simulink model "WF_onshore"  (R2024a)
settings: Solver=VariableStepAuto  StartTime=0  StopTime=0.9  RelTol=1e-3
values from neighbouring files (symbols this model uses):
  cvtr = initialize_NR_VSC_GF(cvtr)    [NR_steadystate_VSC_GF.m]    (also in WF_onshore_SSO_GFL.m = setfield(cvtr,'parameters', p_vary.name,p_vary.val(i)); WF_physical_param_offshore_supersynchronous.m = setfield(cvtr,'parameters', p_vary.name,p_vary.val(i)); WF_physical_param_onshore_SSO_020625.m = setfield(cvtr,'parameters', p_vary.name,p_vary.val(i)); impedance_WT_blackbox.m = base_values(cvtr))
  cvtr1 = cvtr_agg    [WF_physical_param_onshore_SSO_020625.m]
  enable_pll = 1    [impedance_WT_agg.m]    (also in initialize_WT_agg.m; initialize_WT_default_gfl.m; initialize_WT_default_offshore_super.m)
  f1 = 50    [WF_onshore_SSO_GFL.m]    (also in WF_physical_param_offshore_supersynchronous.m; WF_physical_param_onshore_SSO_020625.m; initialize_params_agg.m)
  i = 1    [WF_physical_param_offshore_supersynchronous.m]    (also in WF_physical_param_onshore_SSO_020625.m)
  L = inv(R)    [participation_factors_VSC_GF.m]
  l_OH = 0.2    [WF_onshore_SSO_GFL.m]    (also in WF_physical_param_offshore_supersynchronous.m = 0.1; WF_physical_param_onshore_SSO_020625.m = 0.1; initialize_params_agg.m = 0.1)
  l_tf_wf = tf_params(2,2)    [IM_WF_agg.m]    (also in WF_onshore_SSO_GFL.m = 0.05; WF_physical_param_offshore_supersynchronous.m = 0.05; WF_physical_param_onshore_SSO_020625.m = 0.05; initialize_params_agg.m = 0.05)
  l_tf_wt = tf_params(1,2)    [IM_WF_agg.m]    (also in WF_onshore_SSO_GFL.m = 0.0392; WF_physical_param_offshore_supersynchronous.m = 0.0392; WF_physical_param_onshore_SSO_020625.m = 0.0392; initialize_params_agg.m = 0.0392)
  Lg = p_vary(i)*((Z_b_G/(2*pi*f1)))    [WF_onshore_SSO_GFL.m]    (also in WF_physical_param_offshore_supersynchronous.m; WF_physical_param_onshore_SSO_020625.m; initialize_params_agg.m = 0.1*((Z_b_G/(2*pi*f1))))
  Lg1 = Lg    [WF_physical_param_offshore_supersynchronous.m]    (also in WF_physical_param_onshore_SSO_020625.m)
  Lg2 = Lg    [WF_physical_param_offshore_supersynchronous.m]    (also in WF_physical_param_onshore_SSO_020625.m)
  r_OH = 0.02    [WF_onshore_SSO_GFL.m]    (also in WF_physical_param_offshore_supersynchronous.m = 0.01; WF_physical_param_onshore_SSO_020625.m = 0.01; initialize_params_agg.m)
  r_tf_wf = tf_params(2,1)    [IM_WF_agg.m]    (also in WF_onshore_SSO_GFL.m = 0.005; WF_physical_param_offshore_supersynchronous.m = 0.005; WF_physical_param_onshore_SSO_020625.m = 0.005; initialize_params_agg.m = 0.005)
  r_tf_wt = tf_params(1,1)    [IM_WF_agg.m]    (also in WF_onshore_SSO_GFL.m = 0.0056; WF_physical_param_offshore_supersynchronous.m = 0.0056; WF_physical_param_onshore_SSO_020625.m = 0.0056; initialize_params_agg.m = 0.0056)
  Rg = rg*Z_b_G    [WF_onshore_SSO_GFL.m]    (also in WF_physical_param_offshore_supersynchronous.m; WF_physical_param_onshore_SSO_020625.m; initialize_params_agg.m = 0.01*Z_b_G)
  Sb_WF = (3*1)*5e6    (= 15000000)    [WF_onshore_SSO_GFL.m]    (also in WF_physical_param_offshore_supersynchronous.m; WF_physical_param_onshore_SSO_020625.m; impedance_WT_blackbox.m = n_t*Sb_WT; initialize_params_agg.m = 1000000000)
  Sb_WT = 5e6    (= 5000000)    [IM_WF.m]    (also in WF_onshore_SSO_GFL.m; WF_physical_param_offshore_supersynchronous.m; WF_physical_param_onshore_SSO_020625.m; initialize_params_agg.m)
  selector_current_reference = 3    [impedance_WT_agg.m]    (also in initialize_WT_agg.m; initialize_WT_default_gfl.m; initialize_WT_default_offshore_super.m)
  selector_omega_reference = 1    [impedance_WT_agg.m]    (also in initialize_WT_agg.m; initialize_WT_default_gfl.m; initialize_WT_default_offshore_super.m)
  V_coll = 33e3    (= 33000)    [WF_onshore_SSO_GFL.m]    (also in WF_physical_param_offshore_supersynchronous.m; WF_physical_param_onshore_SSO_020625.m; initialize_params_agg.m)
  V_trans = 220e3    (= 220000)    [WF_onshore_SSO_GFL.m]    (also in WF_physical_param_offshore_supersynchronous.m; WF_physical_param_onshore_SSO_020625.m; initialize_params_agg.m)
  Z_b_G = (V_trans/sqrt(3/2))^2/Sb_WF    [WF_onshore_SSO_GFL.m]    (also in WF_physical_param_offshore_supersynchronous.m = (V_b_trans)^2/Sb_WF; WF_physical_param_onshore_SSO_020625.m = (V_b_trans)^2/Sb_WF; initialize_params_agg.m = (V_b_trans)^2/Sb_WF)
undefined symbols (not defined in the file or in its folder): opts, R
libraries: simulink_extras x104, spsSeriesRLCBranchLib x90, simulink x52, spsThreePhaseVIMeasurementLib x42, spsControlledVoltageSourceLib x42, spsGroundLib x27, spsThreePhaseTransformerTwoWindingsLib x14, powerlib_extras x13, spsVariableInductorLib x6, spsPower3phInstantaneousLib x3, spspowerguiLib x1
(part 2 of 12)

== system WF_onshore/WT_MF3 ==
  Control System : Subsystem  mask{Ts_control=cvtr.parameters.T_cont}
      mask prompts: Ts_control "Sample Time"
  Gain5 : Gain  Gain=cvtr.pu.Vb
  Inverse Park1 : Subsystem
  Subsystem1 : Subsystem
  Subsystem6 : Subsystem
  Three-Phase Transformer (Two Windings) : spsThreePhaseTransformerTwoWindingsLib/Three-Phase Transformer (Two Windings)  Winding1Connection=Yg  Winding2Connection=Yg  CoreType=Three single-phase transformers  SetSaturation=off  Hysteresis=off  DataFile='hysteresis'  SetInitialFlux=off  Measurements=None  UNITS=pu  NominalPower=[Sb_WT, f1 ]  Winding1=[ cvtr.parameters.Vnr ,r_tf_wt/2 , l_tf_wt/2]  Winding2=[ V_coll , r_tf_wt/2, l_tf_wt/2]  Rm=5000  Lm=0  L0=0.5  Saturation=[ 0,0 ; 0.0024,1.2 ; 1.0,1.52 ]  InitialFluxes=[ 0.8 , -0.8 , 0.7 ]  BreakLoop=off  DiscreteSolver=Trapezoidal iterative  DataType=off  TransfoNumber=1
  Three-Phase V-I Measurement : spsThreePhaseVIMeasurementLib/Three-Phase V-I Measurement  VoltageMeasurement=phase-to-ground  SetLabelV=off  LabelV=Vabc  Vpu=off  VpuLL=off  CurrentMeasurement=yes  SetLabelI=off  LabelI=Iabc  Ipu=off  Pbase=100e6  Vbase=500e3  OutputType=Complex  PhasorSimulation=off  PSBequivalent=0
  Transformations (pu and dq) : Subsystem
  filter capacitance1 : Subsystem
      settings: PortSchema="{\"entries\":[{\"content\":{\"sides\":[{\"content\":{\"connectorIds\":[\"LConn1\",\"LConn2\",\"LConn3\"]},\"type\":\"ConnectorPlacement.EquallySpacedRectSide\",\"uuid\":\"e81be3d5-6303-4565-8ca3-afc618f21d70\"},{\"content\":{\"connectorIds\":[],\"side\":\"RIGHT\"},\"type\":\"ConnectorPlacement.EquallySpacedRectSide\",\"uuid\":\"458d9030-e614-487d-87de-3e53be7c7da4\"},{\"content\":{\"connectorIds\":[],\"side\":\"TOP\"},\"type\":\"ConnectorPlacement.EquallySpacedRectSide\",\"uuid\":\"a29d66a0-f095-498d-bb9b-96c7f47699d3\"},{\"content\":{\"connectorIds\":[\"Out1\"],\"side\":\"BOTTOM\"},\"type\":\"ConnectorPlacement.EquallySpacedRectSide\",\"uuid\":\"afc68874-c098-43f5-9b37-53a3b484513b\"}]},\"type\":\"ConnectorPlacement.EquallySpacedConnector\",\"uuid\":\"37f495dd-1c12-4bb8-af72-7ef46bbd951c\"}],\"packageUris\":[\"http://schema.mathworks.com/mf0/Connector/R2020b\"],\"version\":\"1.0\"}"
  filter inductance1 : Subsystem
      settings: PortSchema="{\"entries\":[{\"content\":{\"sides\":[{\"content\":{\"connectorIds\":[\"LConn1\",\"LConn2\",\"LConn3\"]},\"type\":\"ConnectorPlacement.EquallySpacedRectSide\",\"uuid\":\"d3d60048-9578-4fa3-8d11-9c8a66a4b1f9\"},{\"content\":{\"connectorIds\":[\"RConn1\",\"RConn2\",\"RConn3\"],\"side\":\"RIGHT\"},\"type\":\"ConnectorPlacement.EquallySpacedRectSide\",\"uuid\":\"184a2c1d-36ab-46d1-99e4-db01aa31ec94\"},{\"content\":{\"connectorIds\":[\"Out1\"],\"side\":\"TOP\"},\"type\":\"ConnectorPlacement.EquallySpacedRectSide\",\"uuid\":\"db651021-9d7f-4124-8d21-ede853163467\"}]},\"type\":\"ConnectorPlacement.EquallySpacedConnector\",\"uuid\":\"723d0964-19fd-4dbe-91e3-e4ea0bb1cca9\"}],\"packageUris\":[\"http://schema.mathworks.com/mf0/Connector/R2020b\"],\"version\":\"1.0\"}"
  a : PMIOPort  Side=Right
  b : PMIOPort  Port=2  Side=Right
  c : PMIOPort  Port=3  Side=Right
  wires:
  Control System/2(thetavsm) -> [Thetavsm]
  Control System/3(vir) -> [vir]
  Control System/1(thetapll) -> [Thetapll]
  Transformations (pu and dq)/2(il) -> Control System/2(il)  "il"
  Transformations (pu and dq)/1(io) -> Control System/1(io)  "io"
  Transformations (pu and dq)/3(p) -> Control System/3(p)  "p"
  Transformations (pu and dq)/4(q) -> Control System/4(q)  "q"
  Transformations (pu and dq)/5(vo_pll) -> Control System/5(vo_pll)  "vo_pll"
  Transformations (pu and dq)/6(vo) -> Control System/6(vo)  "vo"
  [Thetavsm] -> Transformations (pu and dq)/5(Thetavsm)
  [Thetapll] -> Transformations (pu and dq)/6(Thetapll)
  [vir] -> Gain5/1
  Subsystem6/1(x_dq) -> Inverse Park1/1(x_dq)
  Gain5/1 -> Subsystem6/1(x_d+ix_q)
  Three-Phase V-I Measurement/2 -> [i_abc_grid]  "i_abc_grid"
  Inverse Park1/1(x_abc) -> Subsystem1/1(v_abc)
  Three-Phase V-I Measurement/1 -> [v_abc_grid]  "v_abc_grid"
  [Thetavsm] -> Inverse Park1/2(delta)
  filter capacitance1/1(v_abc) -> [v_abc_filt]  "v_abc_filt"
  filter inductance1/1(i_abc) -> [i_abc_filt]  "i_abc_filt"
  [v_abc_grid] -> Transformations (pu and dq)/3(v_abc_grid)
  [v_abc_filt] -> Transformations (pu and dq)/4(v_abc_filt)
  [i_abc_filt] -> Transformations (pu and dq)/2(i_abc_filt)
  [i_abc_grid] -> Transformations (pu and dq)/1(i_abc_grid)
  connections:
  filter inductance1/RConn3 -- filter capacitance1/LConn3 -- Three-Phase V-I Measurement/LConn3
  filter inductance1/RConn1 -- filter capacitance1/LConn1 -- Three-Phase V-I Measurement/LConn1
  filter inductance1/RConn2 -- filter capacitance1/LConn2 -- Three-Phase V-I Measurement/LConn2
  Subsystem1/RConn1 -- filter inductance1/LConn1
  Subsystem1/RConn2 -- filter inductance1/LConn2
  Subsystem1/RConn3 -- filter inductance1/LConn3
  Three-Phase Transformer (Two Windings)/RConn1 -- a/RConn1
  Three-Phase Transformer (Two Windings)/RConn2 -- b/RConn1
  Three-Phase Transformer (Two Windings)/RConn3 -- c/RConn1
  Three-Phase Transformer (Two Windings)/LConn1 -- Three-Phase V-I Measurement/RConn1
  Three-Phase Transformer (Two Windings)/LConn2 -- Three-Phase V-I Measurement/RConn2
  Three-Phase Transformer (Two Windings)/LConn3 -- Three-Phase V-I Measurement/RConn3

== system WF_onshore/WT_MF4 ==
  Control System : Subsystem  mask{Ts_control=cvtr.parameters.T_cont}
      mask prompts: Ts_control "Sample Time"
  Gain5 : Gain  Gain=cvtr.pu.Vb
  Inverse Park1 : Subsystem
  Subsystem1 : Subsystem
  Subsystem6 : Subsystem
  Three-Phase Transformer (Two Windings) : spsThreePhaseTransformerTwoWindingsLib/Three-Phase Transformer (Two Windings)  Winding1Connection=Yg  Winding2Connection=Yg  CoreType=Three single-phase transformers  SetSaturation=off  Hysteresis=off  DataFile='hysteresis'  SetInitialFlux=off  Measurements=None  UNITS=pu  NominalPower=[Sb_WT, f1 ]  Winding1=[ cvtr.parameters.Vnr ,r_tf_wt/2 , l_tf_wt/2]  Winding2=[ V_coll , r_tf_wt/2, l_tf_wt/2]  Rm=5000  Lm=0  L0=0.5  Saturation=[ 0,0 ; 0.0024,1.2 ; 1.0,1.52 ]  InitialFluxes=[ 0.8 , -0.8 , 0.7 ]  BreakLoop=off  DiscreteSolver=Trapezoidal iterative  DataType=off  TransfoNumber=1
  Three-Phase V-I Measurement : spsThreePhaseVIMeasurementLib/Three-Phase V-I Measurement  VoltageMeasurement=phase-to-ground  SetLabelV=off  LabelV=Vabc  Vpu=off  VpuLL=off  CurrentMeasurement=yes  SetLabelI=off  LabelI=Iabc  Ipu=off  Pbase=100e6  Vbase=500e3  OutputType=Complex  PhasorSimulation=off  PSBequivalent=0
  Transformations (pu and dq) : Subsystem
  filter capacitance1 : Subsystem
      settings: PortSchema="{\"entries\":[{\"content\":{\"sides\":[{\"content\":{\"connectorIds\":[\"LConn1\",\"LConn2\",\"LConn3\"]},\"type\":\"ConnectorPlacement.EquallySpacedRectSide\",\"uuid\":\"e81be3d5-6303-4565-8ca3-afc618f21d70\"},{\"content\":{\"connectorIds\":[],\"side\":\"RIGHT\"},\"type\":\"ConnectorPlacement.EquallySpacedRectSide\",\"uuid\":\"458d9030-e614-487d-87de-3e53be7c7da4\"},{\"content\":{\"connectorIds\":[],\"side\":\"TOP\"},\"type\":\"ConnectorPlacement.EquallySpacedRectSide\",\"uuid\":\"a29d66a0-f095-498d-bb9b-96c7f47699d3\"},{\"content\":{\"connectorIds\":[\"Out1\"],\"side\":\"BOTTOM\"},\"type\":\"ConnectorPlacement.EquallySpacedRectSide\",\"uuid\":\"afc68874-c098-43f5-9b37-53a3b484513b\"}]},\"type\":\"ConnectorPlacement.EquallySpacedConnector\",\"uuid\":\"37f495dd-1c12-4bb8-af72-7ef46bbd951c\"}],\"packageUris\":[\"http://schema.mathworks.com/mf0/Connector/R2020b\"],\"version\":\"1.0\"}"
  filter inductance1 : Subsystem
      settings: PortSchema="{\"entries\":[{\"content\":{\"sides\":[{\"content\":{\"connectorIds\":[\"LConn1\",\"LConn2\",\"LConn3\"]},\"type\":\"ConnectorPlacement.EquallySpacedRectSide\",\"uuid\":\"d3d60048-9578-4fa3-8d11-9c8a66a4b1f9\"},{\"content\":{\"connectorIds\":[\"RConn1\",\"RConn2\",\"RConn3\"],\"side\":\"RIGHT\"},\"type\":\"ConnectorPlacement.EquallySpacedRectSide\",\"uuid\":\"184a2c1d-36ab-46d1-99e4-db01aa31ec94\"},{\"content\":{\"connectorIds\":[\"Out1\"],\"side\":\"TOP\"},\"type\":\"ConnectorPlacement.EquallySpacedRectSide\",\"uuid\":\"db651021-9d7f-4124-8d21-ede853163467\"}]},\"type\":\"ConnectorPlacement.EquallySpacedConnector\",\"uuid\":\"723d0964-19fd-4dbe-91e3-e4ea0bb1cca9\"}],\"packageUris\":[\"http://schema.mathworks.com/mf0/Connector/R2020b\"],\"version\":\"1.0\"}"
  a : PMIOPort  Side=Right
  b : PMIOPort  Port=2  Side=Right
  c : PMIOPort  Port=3  Side=Right
  wires:
  [i_abc_grid] -> Transformations (pu and dq)/1(i_abc_grid)
  [i_abc_filt] -> Transformations (pu and dq)/2(i_abc_filt)
  [v_abc_filt] -> Transformations (pu and dq)/4(v_abc_filt)
  [v_abc_grid] -> Transformations (pu and dq)/3(v_abc_grid)
  filter inductance1/1(i_abc) -> [i_abc_filt]  "i_abc_filt"
  filter capacitance1/1(v_abc) -> [v_abc_filt]  "v_abc_filt"
  [Thetavsm] -> Inverse Park1/2(delta)
  Three-Phase V-I Measurement/1 -> [v_abc_grid]  "v_abc_grid"
  Inverse Park1/1(x_abc) -> Subsystem1/1(v_abc)
  Three-Phase V-I Measurement/2 -> [i_abc_grid]  "i_abc_grid"
  Gain5/1 -> Subsystem6/1(x_d+ix_q)
  Subsystem6/1(x_dq) -> Inverse Park1/1(x_dq)
  [vir] -> Gain5/1
  [Thetapll] -> Transformations (pu and dq)/6(Thetapll)
  [Thetavsm] -> Transformations (pu and dq)/5(Thetavsm)
  Transformations (pu and dq)/6(vo) -> Control System/6(vo)  "vo"
  Transformations (pu and dq)/5(vo_pll) -> Control System/5(vo_pll)  "vo_pll"
  Transformations (pu and dq)/4(q) -> Control System/4(q)  "q"
  Transformations (pu and dq)/3(p) -> Control System/3(p)  "p"
  Transformations (pu and dq)/1(io) -> Control System/1(io)  "io"
  Transformations (pu and dq)/2(il) -> Control System/2(il)  "il"
  Control System/1(thetapll) -> [Thetapll]
  Control System/3(vir) -> [vir]
  Control System/2(thetavsm) -> [Thetavsm]
  connections:
  Three-Phase Transformer (Two Windings)/LConn3 -- Three-Phase V-I Measurement/RConn3
  Three-Phase Transformer (Two Windings)/LConn2 -- Three-Phase V-I Measurement/RConn2
  Three-Phase Transformer (Two Windings)/LConn1 -- Three-Phase V-I Measurement/RConn1
  Three-Phase Transformer (Two Windings)/RConn3 -- c/RConn1
  Three-Phase Transformer (Two Windings)/RConn2 -- b/RConn1
  Three-Phase Transformer (Two Windings)/RConn1 -- a/RConn1
  Subsystem1/RConn3 -- filter inductance1/LConn3
  Subsystem1/RConn2 -- filter inductance1/LConn2
  Subsystem1/RConn1 -- filter inductance1/LConn1
  Three-Phase V-I Measurement/LConn2 -- filter capacitance1/LConn2 -- filter inductance1/RConn2
  Three-Phase V-I Measurement/LConn1 -- filter capacitance1/LConn1 -- filter inductance1/RConn1
  Three-Phase V-I Measurement/LConn3 -- filter capacitance1/LConn3 -- filter inductance1/RConn3

== system WF_onshore/WT_MF5 ==
  Control System : Subsystem  mask{Ts_control=cvtr.parameters.T_cont}
      mask prompts: Ts_control "Sample Time"
  Gain5 : Gain  Gain=cvtr.pu.Vb
  Inverse Park1 : Subsystem
  Subsystem1 : Subsystem
  Subsystem6 : Subsystem
  Three-Phase Transformer (Two Windings) : spsThreePhaseTransformerTwoWindingsLib/Three-Phase Transformer (Two Windings)  Winding1Connection=Yg  Winding2Connection=Yg  CoreType=Three single-phase transformers  SetSaturation=off  Hysteresis=off  DataFile='hysteresis'  SetInitialFlux=off  Measurements=None  UNITS=pu  NominalPower=[Sb_WT, f1 ]  Winding1=[ cvtr.parameters.Vnr ,r_tf_wt/2 , l_tf_wt/2]  Winding2=[ V_coll , r_tf_wt/2, l_tf_wt/2]  Rm=5000  Lm=0  L0=0.5  Saturation=[ 0,0 ; 0.0024,1.2 ; 1.0,1.52 ]  InitialFluxes=[ 0.8 , -0.8 , 0.7 ]  BreakLoop=off  DiscreteSolver=Trapezoidal iterative  DataType=off  TransfoNumber=1
  Three-Phase V-I Measurement : spsThreePhaseVIMeasurementLib/Three-Phase V-I Measurement  VoltageMeasurement=phase-to-ground  SetLabelV=off  LabelV=Vabc  Vpu=off  VpuLL=off  CurrentMeasurement=yes  SetLabelI=off  LabelI=Iabc  Ipu=off  Pbase=100e6  Vbase=500e3  OutputType=Complex  PhasorSimulation=off  PSBequivalent=0
  Transformations (pu and dq) : Subsystem
  filter capacitance1 : Subsystem
      settings: PortSchema="{\"entries\":[{\"content\":{\"sides\":[{\"content\":{\"connectorIds\":[\"LConn1\",\"LConn2\",\"LConn3\"]},\"type\":\"ConnectorPlacement.EquallySpacedRectSide\",\"uuid\":\"e81be3d5-6303-4565-8ca3-afc618f21d70\"},{\"content\":{\"connectorIds\":[],\"side\":\"RIGHT\"},\"type\":\"ConnectorPlacement.EquallySpacedRectSide\",\"uuid\":\"458d9030-e614-487d-87de-3e53be7c7da4\"},{\"content\":{\"connectorIds\":[],\"side\":\"TOP\"},\"type\":\"ConnectorPlacement.EquallySpacedRectSide\",\"uuid\":\"a29d66a0-f095-498d-bb9b-96c7f47699d3\"},{\"content\":{\"connectorIds\":[\"Out1\"],\"side\":\"BOTTOM\"},\"type\":\"ConnectorPlacement.EquallySpacedRectSide\",\"uuid\":\"afc68874-c098-43f5-9b37-53a3b484513b\"}]},\"type\":\"ConnectorPlacement.EquallySpacedConnector\",\"uuid\":\"37f495dd-1c12-4bb8-af72-7ef46bbd951c\"}],\"packageUris\":[\"http://schema.mathworks.com/mf0/Connector/R2020b\"],\"version\":\"1.0\"}"
  filter inductance1 : Subsystem
      settings: PortSchema="{\"entries\":[{\"content\":{\"sides\":[{\"content\":{\"connectorIds\":[\"LConn1\",\"LConn2\",\"LConn3\"]},\"type\":\"ConnectorPlacement.EquallySpacedRectSide\",\"uuid\":\"d3d60048-9578-4fa3-8d11-9c8a66a4b1f9\"},{\"content\":{\"connectorIds\":[\"RConn1\",\"RConn2\",\"RConn3\"],\"side\":\"RIGHT\"},\"type\":\"ConnectorPlacement.EquallySpacedRectSide\",\"uuid\":\"184a2c1d-36ab-46d1-99e4-db01aa31ec94\"},{\"content\":{\"connectorIds\":[\"Out1\"],\"side\":\"TOP\"},\"type\":\"ConnectorPlacement.EquallySpacedRectSide\",\"uuid\":\"db651021-9d7f-4124-8d21-ede853163467\"}]},\"type\":\"ConnectorPlacement.EquallySpacedConnector\",\"uuid\":\"723d0964-19fd-4dbe-91e3-e4ea0bb1cca9\"}],\"packageUris\":[\"http://schema.mathworks.com/mf0/Connector/R2020b\"],\"version\":\"1.0\"}"
  a : PMIOPort  Side=Right
  b : PMIOPort  Port=2  Side=Right
  c : PMIOPort  Port=3  Side=Right
  wires:
  Control System/2(thetavsm) -> [Thetavsm]
  Control System/3(vir) -> [vir]
  Control System/1(thetapll) -> [Thetapll]
  Transformations (pu and dq)/2(il) -> Control System/2(il)  "il"
  Transformations (pu and dq)/1(io) -> Control System/1(io)  "io"
  Transformations (pu and dq)/3(p) -> Control System/3(p)  "p"
  Transformations (pu and dq)/4(q) -> Control System/4(q)  "q"
  Transformations (pu and dq)/5(vo_pll) -> Control System/5(vo_pll)  "vo_pll"
  Transformations (pu and dq)/6(vo) -> Control System/6(vo)  "vo"
  [Thetavsm] -> Transformations (pu and dq)/5(Thetavsm)
  [Thetapll] -> Transformations (pu and dq)/6(Thetapll)
  [vir] -> Gain5/1
  Subsystem6/1(x_dq) -> Inverse Park1/1(x_dq)
  Gain5/1 -> Subsystem6/1(x_d+ix_q)
  Three-Phase V-I Measurement/2 -> [i_abc_grid]  "i_abc_grid"
  Inverse Park1/1(x_abc) -> Subsystem1/1(v_abc)
  Three-Phase V-I Measurement/1 -> [v_abc_grid]  "v_abc_grid"
  [Thetavsm] -> Inverse Park1/2(delta)
  filter capacitance1/1(v_abc) -> [v_abc_filt]  "v_abc_filt"
  filter inductance1/1(i_abc) -> [i_abc_filt]  "i_abc_filt"
  [v_abc_grid] -> Transformations (pu and dq)/3(v_abc_grid)
  [v_abc_filt] -> Transformations (pu and dq)/4(v_abc_filt)
  [i_abc_filt] -> Transformations (pu and dq)/2(i_abc_filt)
  [i_abc_grid] -> Transformations (pu and dq)/1(i_abc_grid)
  connections:
  filter inductance1/RConn3 -- filter capacitance1/LConn3 -- Three-Phase V-I Measurement/LConn3
  filter inductance1/RConn1 -- filter capacitance1/LConn1 -- Three-Phase V-I Measurement/LConn1
  filter inductance1/RConn2 -- filter capacitance1/LConn2 -- Three-Phase V-I Measurement/LConn2
  Subsystem1/RConn1 -- filter inductance1/LConn1
  Subsystem1/RConn2 -- filter inductance1/LConn2
  Subsystem1/RConn3 -- filter inductance1/LConn3
  Three-Phase Transformer (Two Windings)/RConn1 -- a/RConn1
  Three-Phase Transformer (Two Windings)/RConn2 -- b/RConn1
  Three-Phase Transformer (Two Windings)/RConn3 -- c/RConn1
  Three-Phase Transformer (Two Windings)/LConn1 -- Three-Phase V-I Measurement/RConn1
  Three-Phase Transformer (Two Windings)/LConn2 -- Three-Phase V-I Measurement/RConn2
  Three-Phase Transformer (Two Windings)/LConn3 -- Three-Phase V-I Measurement/RConn3

== system WF_onshore/WT_MF6 ==
  Control System : Subsystem  mask{Ts_control=cvtr.parameters.T_cont}
      mask prompts: Ts_control "Sample Time"
  Gain5 : Gain  Gain=cvtr.pu.Vb
  Inverse Park1 : Subsystem
  Subsystem1 : Subsystem
  Subsystem6 : Subsystem
  Three-Phase Transformer (Two Windings) : spsThreePhaseTransformerTwoWindingsLib/Three-Phase Transformer (Two Windings)  Winding1Connection=Yg  Winding2Connection=Yg  CoreType=Three single-phase transformers  SetSaturation=off  Hysteresis=off  DataFile='hysteresis'  SetInitialFlux=off  Measurements=None  UNITS=pu  NominalPower=[Sb_WT, f1 ]  Winding1=[ cvtr.parameters.Vnr ,r_tf_wt/2 , l_tf_wt/2]  Winding2=[ V_coll , r_tf_wt/2, l_tf_wt/2]  Rm=5000  Lm=0  L0=0.5  Saturation=[ 0,0 ; 0.0024,1.2 ; 1.0,1.52 ]  InitialFluxes=[ 0.8 , -0.8 , 0.7 ]  BreakLoop=off  DiscreteSolver=Trapezoidal iterative  DataType=off  TransfoNumber=1
  Three-Phase V-I Measurement : spsThreePhaseVIMeasurementLib/Three-Phase V-I Measurement  VoltageMeasurement=phase-to-ground  SetLabelV=off  LabelV=Vabc  Vpu=off  VpuLL=off  CurrentMeasurement=yes  SetLabelI=off  LabelI=Iabc  Ipu=off  Pbase=100e6  Vbase=500e3  OutputType=Complex  PhasorSimulation=off  PSBequivalent=0
  Transformations (pu and dq) : Subsystem
  filter capacitance1 : Subsystem
      settings: PortSchema="{\"entries\":[{\"content\":{\"sides\":[{\"content\":{\"connectorIds\":[\"LConn1\",\"LConn2\",\"LConn3\"]},\"type\":\"ConnectorPlacement.EquallySpacedRectSide\",\"uuid\":\"e81be3d5-6303-4565-8ca3-afc618f21d70\"},{\"content\":{\"connectorIds\":[],\"side\":\"RIGHT\"},\"type\":\"ConnectorPlacement.EquallySpacedRectSide\",\"uuid\":\"458d9030-e614-487d-87de-3e53be7c7da4\"},{\"content\":{\"connectorIds\":[],\"side\":\"TOP\"},\"type\":\"ConnectorPlacement.EquallySpacedRectSide\",\"uuid\":\"a29d66a0-f095-498d-bb9b-96c7f47699d3\"},{\"content\":{\"connectorIds\":[\"Out1\"],\"side\":\"BOTTOM\"},\"type\":\"ConnectorPlacement.EquallySpacedRectSide\",\"uuid\":\"afc68874-c098-43f5-9b37-53a3b484513b\"}]},\"type\":\"ConnectorPlacement.EquallySpacedConnector\",\"uuid\":\"37f495dd-1c12-4bb8-af72-7ef46bbd951c\"}],\"packageUris\":[\"http://schema.mathworks.com/mf0/Connector/R2020b\"],\"version\":\"1.0\"}"
  filter inductance1 : Subsystem
      settings: PortSchema="{\"entries\":[{\"content\":{\"sides\":[{\"content\":{\"connectorIds\":[\"LConn1\",\"LConn2\",\"LConn3\"]},\"type\":\"ConnectorPlacement.EquallySpacedRectSide\",\"uuid\":\"d3d60048-9578-4fa3-8d11-9c8a66a4b1f9\"},{\"content\":{\"connectorIds\":[\"RConn1\",\"RConn2\",\"RConn3\"],\"side\":\"RIGHT\"},\"type\":\"ConnectorPlacement.EquallySpacedRectSide\",\"uuid\":\"184a2c1d-36ab-46d1-99e4-db01aa31ec94\"},{\"content\":{\"connectorIds\":[\"Out1\"],\"side\":\"TOP\"},\"type\":\"ConnectorPlacement.EquallySpacedRectSide\",\"uuid\":\"db651021-9d7f-4124-8d21-ede853163467\"}]},\"type\":\"ConnectorPlacement.EquallySpacedConnector\",\"uuid\":\"723d0964-19fd-4dbe-91e3-e4ea0bb1cca9\"}],\"packageUris\":[\"http://schema.mathworks.com/mf0/Connector/R2020b\"],\"version\":\"1.0\"}"
  a : PMIOPort  Side=Right
  b : PMIOPort  Port=2  Side=Right
  c : PMIOPort  Port=3  Side=Right
  wires:
  [i_abc_grid] -> Transformations (pu and dq)/1(i_abc_grid)
  [i_abc_filt] -> Transformations (pu and dq)/2(i_abc_filt)
  [v_abc_filt] -> Transformations (pu and dq)/4(v_abc_filt)
  [v_abc_grid] -> Transformations (pu and dq)/3(v_abc_grid)
  filter inductance1/1(i_abc) -> [i_abc_filt]  "i_abc_filt"
  filter capacitance1/1(v_abc) -> [v_abc_filt]  "v_abc_filt"
  [Thetavsm] -> Inverse Park1/2(delta)
  Three-Phase V-I Measurement/1 -> [v_abc_grid]  "v_abc_grid"
  Inverse Park1/1(x_abc) -> Subsystem1/1(v_abc)
  Three-Phase V-I Measurement/2 -> [i_abc_grid]  "i_abc_grid"
  Gain5/1 -> Subsystem6/1(x_d+ix_q)
  Subsystem6/1(x_dq) -> Inverse Park1/1(x_dq)
  [vir] -> Gain5/1
  [Thetapll] -> Transformations (pu and dq)/6(Thetapll)
  [Thetavsm] -> Transformations (pu and dq)/5(Thetavsm)
  Transformations (pu and dq)/6(vo) -> Control System/6(vo)  "vo"
  Transformations (pu and dq)/5(vo_pll) -> Control System/5(vo_pll)  "vo_pll"
  Transformations (pu and dq)/4(q) -> Control System/4(q)  "q"
  Transformations (pu and dq)/3(p) -> Control System/3(p)  "p"
  Transformations (pu and dq)/1(io) -> Control System/1(io)  "io"
  Transformations (pu and dq)/2(il) -> Control System/2(il)  "il"
  Control System/1(thetapll) -> [Thetapll]
  Control System/3(vir) -> [vir]
  Control System/2(thetavsm) -> [Thetavsm]
  connections:
  Three-Phase Transformer (Two Windings)/LConn3 -- Three-Phase V-I Measurement/RConn3
  Three-Phase Transformer (Two Windings)/LConn2 -- Three-Phase V-I Measurement/RConn2
  Three-Phase Transformer (Two Windings)/LConn1 -- Three-Phase V-I Measurement/RConn1
  Three-Phase Transformer (Two Windings)/RConn3 -- c/RConn1
  Three-Phase Transformer (Two Windings)/RConn2 -- b/RConn1
  Three-Phase Transformer (Two Windings)/RConn1 -- a/RConn1
  Subsystem1/RConn3 -- filter inductance1/LConn3
  Subsystem1/RConn2 -- filter inductance1/LConn2
  Subsystem1/RConn1 -- filter inductance1/LConn1
  Three-Phase V-I Measurement/LConn2 -- filter capacitance1/LConn2 -- filter inductance1/RConn2
  Three-Phase V-I Measurement/LConn1 -- filter capacitance1/LConn1 -- filter inductance1/RConn1
  Three-Phase V-I Measurement/LConn3 -- filter capacitance1/LConn3 -- filter inductance1/RConn3

== system WF_onshore/WT_MF7 ==
  Control System : Subsystem  mask{Ts_control=cvtr.parameters.T_cont}
      mask prompts: Ts_control "Sample Time"
  Gain5 : Gain  Gain=cvtr.pu.Vb
  Inverse Park1 : Subsystem
  Subsystem1 : Subsystem
  Subsystem6 : Subsystem
  Three-Phase Transformer (Two Windings) : spsThreePhaseTransformerTwoWindingsLib/Three-Phase Transformer (Two Windings)  Winding1Connection=Yg  Winding2Connection=Yg  CoreType=Three single-phase transformers  SetSaturation=off  Hysteresis=off  DataFile='hysteresis'  SetInitialFlux=off  Measurements=None  UNITS=pu  NominalPower=[Sb_WT, f1 ]  Winding1=[ cvtr.parameters.Vnr ,r_tf_wt/2 , l_tf_wt/2]  Winding2=[ V_coll , r_tf_wt/2, l_tf_wt/2]  Rm=5000  Lm=0  L0=0.5  Saturation=[ 0,0 ; 0.0024,1.2 ; 1.0,1.52 ]  InitialFluxes=[ 0.8 , -0.8 , 0.7 ]  BreakLoop=off  DiscreteSolver=Trapezoidal iterative  DataType=off  TransfoNumber=1
  Three-Phase V-I Measurement : spsThreePhaseVIMeasurementLib/Three-Phase V-I Measurement  VoltageMeasurement=phase-to-ground  SetLabelV=off  LabelV=Vabc  Vpu=off  VpuLL=off  CurrentMeasurement=yes  SetLabelI=off  LabelI=Iabc  Ipu=off  Pbase=100e6  Vbase=500e3  OutputType=Complex  PhasorSimulation=off  PSBequivalent=0
  Transformations (pu and dq) : Subsystem
  filter capacitance1 : Subsystem
      settings: PortSchema="{\"entries\":[{\"content\":{\"sides\":[{\"content\":{\"connectorIds\":[\"LConn1\",\"LConn2\",\"LConn3\"]},\"type\":\"ConnectorPlacement.EquallySpacedRectSide\",\"uuid\":\"e81be3d5-6303-4565-8ca3-afc618f21d70\"},{\"content\":{\"connectorIds\":[],\"side\":\"RIGHT\"},\"type\":\"ConnectorPlacement.EquallySpacedRectSide\",\"uuid\":\"458d9030-e614-487d-87de-3e53be7c7da4\"},{\"content\":{\"connectorIds\":[],\"side\":\"TOP\"},\"type\":\"ConnectorPlacement.EquallySpacedRectSide\",\"uuid\":\"a29d66a0-f095-498d-bb9b-96c7f47699d3\"},{\"content\":{\"connectorIds\":[\"Out1\"],\"side\":\"BOTTOM\"},\"type\":\"ConnectorPlacement.EquallySpacedRectSide\",\"uuid\":\"afc68874-c098-43f5-9b37-53a3b484513b\"}]},\"type\":\"ConnectorPlacement.EquallySpacedConnector\",\"uuid\":\"37f495dd-1c12-4bb8-af72-7ef46bbd951c\"}],\"packageUris\":[\"http://schema.mathworks.com/mf0/Connector/R2020b\"],\"version\":\"1.0\"}"
  filter inductance1 : Subsystem
      settings: PortSchema="{\"entries\":[{\"content\":{\"sides\":[{\"content\":{\"connectorIds\":[\"LConn1\",\"LConn2\",\"LConn3\"]},\"type\":\"ConnectorPlacement.EquallySpacedRectSide\",\"uuid\":\"d3d60048-9578-4fa3-8d11-9c8a66a4b1f9\"},{\"content\":{\"connectorIds\":[\"RConn1\",\"RConn2\",\"RConn3\"],\"side\":\"RIGHT\"},\"type\":\"ConnectorPlacement.EquallySpacedRectSide\",\"uuid\":\"184a2c1d-36ab-46d1-99e4-db01aa31ec94\"},{\"content\":{\"connectorIds\":[\"Out1\"],\"side\":\"TOP\"},\"type\":\"ConnectorPlacement.EquallySpacedRectSide\",\"uuid\":\"db651021-9d7f-4124-8d21-ede853163467\"}]},\"type\":\"ConnectorPlacement.EquallySpacedConnector\",\"uuid\":\"723d0964-19fd-4dbe-91e3-e4ea0bb1cca9\"}],\"packageUris\":[\"http://schema.mathworks.com/mf0/Connector/R2020b\"],\"version\":\"1.0\"}"
  a : PMIOPort  Side=Right
  b : PMIOPort  Port=2  Side=Right
  c : PMIOPort  Port=3  Side=Right
  wires:
  Control System/2(thetavsm) -> [Thetavsm]
  Control System/3(vir) -> [vir]
  Control System/1(thetapll) -> [Thetapll]
  Transformations (pu and dq)/2(il) -> Control System/2(il)  "il"
  Transformations (pu and dq)/1(io) -> Control System/1(io)  "io"
  Transformations (pu and dq)/3(p) -> Control System/3(p)  "p"
  Transformations (pu and dq)/4(q) -> Control System/4(q)  "q"
  Transformations (pu and dq)/5(vo_pll) -> Control System/5(vo_pll)  "vo_pll"
  Transformations (pu and dq)/6(vo) -> Control System/6(vo)  "vo"
  [Thetavsm] -> Transformations (pu and dq)/5(Thetavsm)
  [Thetapll] -> Transformations (pu and dq)/6(Thetapll)
  [vir] -> Gain5/1
  Subsystem6/1(x_dq) -> Inverse Park1/1(x_dq)
  Gain5/1 -> Subsystem6/1(x_d+ix_q)
  Three-Phase V-I Measurement/2 -> [i_abc_grid]  "i_abc_grid"
  Inverse Park1/1(x_abc) -> Subsystem1/1(v_abc)
  Three-Phase V-I Measurement/1 -> [v_abc_grid]  "v_abc_grid"
  [Thetavsm] -> Inverse Park1/2(delta)
  filter capacitance1/1(v_abc) -> [v_abc_filt]  "v_abc_filt"
  filter inductance1/1(i_abc) -> [i_abc_filt]  "i_abc_filt"
  [v_abc_grid] -> Transformations (pu and dq)/3(v_abc_grid)
  [v_abc_filt] -> Transformations (pu and dq)/4(v_abc_filt)
  [i_abc_filt] -> Transformations (pu and dq)/2(i_abc_filt)
  [i_abc_grid] -> Transformations (pu and dq)/1(i_abc_grid)
  connections:
  filter inductance1/RConn3 -- filter capacitance1/LConn3 -- Three-Phase V-I Measurement/LConn3
  filter inductance1/RConn1 -- filter capacitance1/LConn1 -- Three-Phase V-I Measurement/LConn1
  filter inductance1/RConn2 -- filter capacitance1/LConn2 -- Three-Phase V-I Measurement/LConn2
  Subsystem1/RConn1 -- filter inductance1/LConn1
  Subsystem1/RConn2 -- filter inductance1/LConn2
  Subsystem1/RConn3 -- filter inductance1/LConn3
  Three-Phase Transformer (Two Windings)/RConn1 -- a/RConn1
  Three-Phase Transformer (Two Windings)/RConn2 -- b/RConn1
  Three-Phase Transformer (Two Windings)/RConn3 -- c/RConn1
  Three-Phase Transformer (Two Windings)/LConn1 -- Three-Phase V-I Measurement/RConn1
  Three-Phase Transformer (Two Windings)/LConn2 -- Three-Phase V-I Measurement/RConn2
  Three-Phase Transformer (Two Windings)/LConn3 -- Three-Phase V-I Measurement/RConn3

== system WF_onshore/WT_MF8 ==
  Control System : Subsystem  mask{Ts_control=cvtr.parameters.T_cont}
      mask prompts: Ts_control "Sample Time"
  Gain5 : Gain  Gain=cvtr.pu.Vb
  Inverse Park1 : Subsystem
  Subsystem1 : Subsystem
  Subsystem6 : Subsystem
  Three-Phase Transformer (Two Windings) : spsThreePhaseTransformerTwoWindingsLib/Three-Phase Transformer (Two Windings)  Winding1Connection=Yg  Winding2Connection=Yg  CoreType=Three single-phase transformers  SetSaturation=off  Hysteresis=off  DataFile='hysteresis'  SetInitialFlux=off  Measurements=None  UNITS=pu  NominalPower=[Sb_WT, f1 ]  Winding1=[ cvtr.parameters.Vnr ,r_tf_wt/2 , l_tf_wt/2]  Winding2=[ V_coll , r_tf_wt/2, l_tf_wt/2]  Rm=5000  Lm=0  L0=0.5  Saturation=[ 0,0 ; 0.0024,1.2 ; 1.0,1.52 ]  InitialFluxes=[ 0.8 , -0.8 , 0.7 ]  BreakLoop=off  DiscreteSolver=Trapezoidal iterative  DataType=off  TransfoNumber=1
  Three-Phase V-I Measurement : spsThreePhaseVIMeasurementLib/Three-Phase V-I Measurement  VoltageMeasurement=phase-to-ground  SetLabelV=off  LabelV=Vabc  Vpu=off  VpuLL=off  CurrentMeasurement=yes  SetLabelI=off  LabelI=Iabc  Ipu=off  Pbase=100e6  Vbase=500e3  OutputType=Complex  PhasorSimulation=off  PSBequivalent=0
  Transformations (pu and dq) : Subsystem
  filter capacitance1 : Subsystem
      settings: PortSchema="{\"entries\":[{\"content\":{\"sides\":[{\"content\":{\"connectorIds\":[\"LConn1\",\"LConn2\",\"LConn3\"]},\"type\":\"ConnectorPlacement.EquallySpacedRectSide\",\"uuid\":\"e81be3d5-6303-4565-8ca3-afc618f21d70\"},{\"content\":{\"connectorIds\":[],\"side\":\"RIGHT\"},\"type\":\"ConnectorPlacement.EquallySpacedRectSide\",\"uuid\":\"458d9030-e614-487d-87de-3e53be7c7da4\"},{\"content\":{\"connectorIds\":[],\"side\":\"TOP\"},\"type\":\"ConnectorPlacement.EquallySpacedRectSide\",\"uuid\":\"a29d66a0-f095-498d-bb9b-96c7f47699d3\"},{\"content\":{\"connectorIds\":[\"Out1\"],\"side\":\"BOTTOM\"},\"type\":\"ConnectorPlacement.EquallySpacedRectSide\",\"uuid\":\"afc68874-c098-43f5-9b37-53a3b484513b\"}]},\"type\":\"ConnectorPlacement.EquallySpacedConnector\",\"uuid\":\"37f495dd-1c12-4bb8-af72-7ef46bbd951c\"}],\"packageUris\":[\"http://schema.mathworks.com/mf0/Connector/R2020b\"],\"version\":\"1.0\"}"
  filter inductance1 : Subsystem
      settings: PortSchema="{\"entries\":[{\"content\":{\"sides\":[{\"content\":{\"connectorIds\":[\"LConn1\",\"LConn2\",\"LConn3\"]},\"type\":\"ConnectorPlacement.EquallySpacedRectSide\",\"uuid\":\"d3d60048-9578-4fa3-8d11-9c8a66a4b1f9\"},{\"content\":{\"connectorIds\":[\"RConn1\",\"RConn2\",\"RConn3\"],\"side\":\"RIGHT\"},\"type\":\"ConnectorPlacement.EquallySpacedRectSide\",\"uuid\":\"184a2c1d-36ab-46d1-99e4-db01aa31ec94\"},{\"content\":{\"connectorIds\":[\"Out1\"],\"side\":\"TOP\"},\"type\":\"ConnectorPlacement.EquallySpacedRectSide\",\"uuid\":\"db651021-9d7f-4124-8d21-ede853163467\"}]},\"type\":\"ConnectorPlacement.EquallySpacedConnector\",\"uuid\":\"723d0964-19fd-4dbe-91e3-e4ea0bb1cca9\"}],\"packageUris\":[\"http://schema.mathworks.com/mf0/Connector/R2020b\"],\"version\":\"1.0\"}"
  a : PMIOPort  Side=Right
  b : PMIOPort  Port=2  Side=Right
  c : PMIOPort  Port=3  Side=Right
  wires:
  [i_abc_grid] -> Transformations (pu and dq)/1(i_abc_grid)
  [i_abc_filt] -> Transformations (pu and dq)/2(i_abc_filt)
  [v_abc_filt] -> Transformations (pu and dq)/4(v_abc_filt)
  [v_abc_grid] -> Transformations (pu and dq)/3(v_abc_grid)
  filter inductance1/1(i_abc) -> [i_abc_filt]  "i_abc_filt"
  filter capacitance1/1(v_abc) -> [v_abc_filt]  "v_abc_filt"
  [Thetavsm] -> Inverse Park1/2(delta)
  Three-Phase V-I Measurement/1 -> [v_abc_grid]  "v_abc_grid"
  Inverse Park1/1(x_abc) -> Subsystem1/1(v_abc)
  Three-Phase V-I Measurement/2 -> [i_abc_grid]  "i_abc_grid"
  Gain5/1 -> Subsystem6/1(x_d+ix_q)
  Subsystem6/1(x_dq) -> Inverse Park1/1(x_dq)
  [vir] -> Gain5/1
  [Thetapll] -> Transformations (pu and dq)/6(Thetapll)
  [Thetavsm] -> Transformations (pu and dq)/5(Thetavsm)
  Transformations (pu and dq)/6(vo) -> Control System/6(vo)  "vo"
  Transformations (pu and dq)/5(vo_pll) -> Control System/5(vo_pll)  "vo_pll"
  Transformations (pu and dq)/4(q) -> Control System/4(q)  "q"
  Transformations (pu and dq)/3(p) -> Control System/3(p)  "p"
  Transformations (pu and dq)/1(io) -> Control System/1(io)  "io"
  Transformations (pu and dq)/2(il) -> Control System/2(il)  "il"
  Control System/1(thetapll) -> [Thetapll]
  Control System/3(vir) -> [vir]
  Control System/2(thetavsm) -> [Thetavsm]
  connections:
  Three-Phase Transformer (Two Windings)/LConn3 -- Three-Phase V-I Measurement/RConn3
  Three-Phase Transformer (Two Windings)/LConn2 -- Three-Phase V-I Measurement/RConn2
  Three-Phase Transformer (Two Windings)/LConn1 -- Three-Phase V-I Measurement/RConn1
  Three-Phase Transformer (Two Windings)/RConn3 -- c/RConn1
  Three-Phase Transformer (Two Windings)/RConn2 -- b/RConn1
  Three-Phase Transformer (Two Windings)/RConn1 -- a/RConn1
  Subsystem1/RConn3 -- filter inductance1/LConn3
  Subsystem1/RConn2 -- filter inductance1/LConn2
  Subsystem1/RConn1 -- filter inductance1/LConn1
  Three-Phase V-I Measurement/LConn2 -- filter capacitance1/LConn2 -- filter inductance1/RConn2
  Three-Phase V-I Measurement/LConn1 -- filter capacitance1/LConn1 -- filter inductance1/RConn1
  Three-Phase V-I Measurement/LConn3 -- filter capacitance1/LConn3 -- filter inductance1/RConn3

== system WF_onshore/WT_MF9 ==
  Control System : Subsystem  mask{Ts_control=cvtr.parameters.T_cont}
      mask prompts: Ts_control "Sample Time"
  Gain5 : Gain  Gain=cvtr.pu.Vb
  Inverse Park1 : Subsystem
  Subsystem1 : Subsystem
  Subsystem6 : Subsystem
  Three-Phase Transformer (Two Windings) : spsThreePhaseTransformerTwoWindingsLib/Three-Phase Transformer (Two Windings)  Winding1Connection=Yg  Winding2Connection=Yg  CoreType=Three single-phase transformers  SetSaturation=off  Hysteresis=off  DataFile='hysteresis'  SetInitialFlux=off  Measurements=None  UNITS=pu  NominalPower=[Sb_WT, f1 ]  Winding1=[ cvtr.parameters.Vnr ,r_tf_wt/2 , l_tf_wt/2]  Winding2=[ V_coll , r_tf_wt/2, l_tf_wt/2]  Rm=5000  Lm=0  L0=0.5  Saturation=[ 0,0 ; 0.0024,1.2 ; 1.0,1.52 ]  InitialFluxes=[ 0.8 , -0.8 , 0.7 ]  BreakLoop=off  DiscreteSolver=Trapezoidal iterative  DataType=off  TransfoNumber=1
  Three-Phase V-I Measurement : spsThreePhaseVIMeasurementLib/Three-Phase V-I Measurement  VoltageMeasurement=phase-to-ground  SetLabelV=off  LabelV=Vabc  Vpu=off  VpuLL=off  CurrentMeasurement=yes  SetLabelI=off  LabelI=Iabc  Ipu=off  Pbase=100e6  Vbase=500e3  OutputType=Complex  PhasorSimulation=off  PSBequivalent=0
  Transformations (pu and dq) : Subsystem
  filter capacitance1 : Subsystem
      settings: PortSchema="{\"entries\":[{\"content\":{\"sides\":[{\"content\":{\"connectorIds\":[\"LConn1\",\"LConn2\",\"LConn3\"]},\"type\":\"ConnectorPlacement.EquallySpacedRectSide\",\"uuid\":\"e81be3d5-6303-4565-8ca3-afc618f21d70\"},{\"content\":{\"connectorIds\":[],\"side\":\"RIGHT\"},\"type\":\"ConnectorPlacement.EquallySpacedRectSide\",\"uuid\":\"458d9030-e614-487d-87de-3e53be7c7da4\"},{\"content\":{\"connectorIds\":[],\"side\":\"TOP\"},\"type\":\"ConnectorPlacement.EquallySpacedRectSide\",\"uuid\":\"a29d66a0-f095-498d-bb9b-96c7f47699d3\"},{\"content\":{\"connectorIds\":[\"Out1\"],\"side\":\"BOTTOM\"},\"type\":\"ConnectorPlacement.EquallySpacedRectSide\",\"uuid\":\"afc68874-c098-43f5-9b37-53a3b484513b\"}]},\"type\":\"ConnectorPlacement.EquallySpacedConnector\",\"uuid\":\"37f495dd-1c12-4bb8-af72-7ef46bbd951c\"}],\"packageUris\":[\"http://schema.mathworks.com/mf0/Connector/R2020b\"],\"version\":\"1.0\"}"
  filter inductance1 : Subsystem
      settings: PortSchema="{\"entries\":[{\"content\":{\"sides\":[{\"content\":{\"connectorIds\":[\"LConn1\",\"LConn2\",\"LConn3\"]},\"type\":\"ConnectorPlacement.EquallySpacedRectSide\",\"uuid\":\"d3d60048-9578-4fa3-8d11-9c8a66a4b1f9\"},{\"content\":{\"connectorIds\":[\"RConn1\",\"RConn2\",\"RConn3\"],\"side\":\"RIGHT\"},\"type\":\"ConnectorPlacement.EquallySpacedRectSide\",\"uuid\":\"184a2c1d-36ab-46d1-99e4-db01aa31ec94\"},{\"content\":{\"connectorIds\":[\"Out1\"],\"side\":\"TOP\"},\"type\":\"ConnectorPlacement.EquallySpacedRectSide\",\"uuid\":\"db651021-9d7f-4124-8d21-ede853163467\"}]},\"type\":\"ConnectorPlacement.EquallySpacedConnector\",\"uuid\":\"723d0964-19fd-4dbe-91e3-e4ea0bb1cca9\"}],\"packageUris\":[\"http://schema.mathworks.com/mf0/Connector/R2020b\"],\"version\":\"1.0\"}"
  a : PMIOPort  Side=Right
  b : PMIOPort  Port=2  Side=Right
  c : PMIOPort  Port=3  Side=Right
  wires:
  Control System/2(thetavsm) -> [Thetavsm]
  Control System/3(vir) -> [vir]
  Control System/1(thetapll) -> [Thetapll]
  Transformations (pu and dq)/2(il) -> Control System/2(il)  "il"
  Transformations (pu and dq)/1(io) -> Control System/1(io)  "io"
  Transformations (pu and dq)/3(p) -> Control System/3(p)  "p"
  Transformations (pu and dq)/4(q) -> Control System/4(q)  "q"
  Transformations (pu and dq)/5(vo_pll) -> Control System/5(vo_pll)  "vo_pll"
  Transformations (pu and dq)/6(vo) -> Control System/6(vo)  "vo"
  [Thetavsm] -> Transformations (pu and dq)/5(Thetavsm)
  [Thetapll] -> Transformations (pu and dq)/6(Thetapll)
  [vir] -> Gain5/1
  Subsystem6/1(x_dq) -> Inverse Park1/1(x_dq)
  Gain5/1 -> Subsystem6/1(x_d+ix_q)
  Three-Phase V-I Measurement/2 -> [i_abc_grid]  "i_abc_grid"
  Inverse Park1/1(x_abc) -> Subsystem1/1(v_abc)
  Three-Phase V-I Measurement/1 -> [v_abc_grid]  "v_abc_grid"
  [Thetavsm] -> Inverse Park1/2(delta)
  filter capacitance1/1(v_abc) -> [v_abc_filt]  "v_abc_filt"
  filter inductance1/1(i_abc) -> [i_abc_filt]  "i_abc_filt"
  [v_abc_grid] -> Transformations (pu and dq)/3(v_abc_grid)
  [v_abc_filt] -> Transformations (pu and dq)/4(v_abc_filt)
  [i_abc_filt] -> Transformations (pu and dq)/2(i_abc_filt)
  [i_abc_grid] -> Transformations (pu and dq)/1(i_abc_grid)
  connections:
  filter inductance1/RConn3 -- filter capacitance1/LConn3 -- Three-Phase V-I Measurement/LConn3
  filter inductance1/RConn1 -- filter capacitance1/LConn1 -- Three-Phase V-I Measurement/LConn1
  filter inductance1/RConn2 -- filter capacitance1/LConn2 -- Three-Phase V-I Measurement/LConn2
  Subsystem1/RConn1 -- filter inductance1/LConn1
  Subsystem1/RConn2 -- filter inductance1/LConn2
  Subsystem1/RConn3 -- filter inductance1/LConn3
  Three-Phase Transformer (Two Windings)/RConn1 -- a/RConn1
  Three-Phase Transformer (Two Windings)/RConn2 -- b/RConn1
  Three-Phase Transformer (Two Windings)/RConn3 -- c/RConn1
  Three-Phase Transformer (Two Windings)/LConn1 -- Three-Phase V-I Measurement/RConn1
  Three-Phase Transformer (Two Windings)/LConn2 -- Three-Phase V-I Measurement/RConn2
  Three-Phase Transformer (Two Windings)/LConn3 -- Three-Phase V-I Measurement/RConn3

== system WF_onshore/VoltageSource/Inverse Park1 ==
  x_dq : Inport
  delta : Inport  Port=2
  Demux1 : Demux  Outputs=2
  Fcn : Fcn  Expr=cos(u(3))*u(1)-sin(u(3))*u(2)
  Fcn1 : Fcn  Expr=cos(u(3)-2/3*pi)*u(1)-sin(u(3)-2/3*pi)*u(2)
  Fcn2 : Fcn  Expr=cos(u(3)+2/3*pi)*u(1)-sin(u(3)+2/3*pi)*u(2)
  Mux : Mux  Inputs=3
  Mux1 : Mux  Inputs=3
  x_abc : Outport
  wires:
  Mux1/1 -> x_abc/1
  Mux/1 -> Fcn1/1, Fcn2/1, Fcn/1
  delta/1 -> Mux/3
  x_dq/1 -> Demux1/1
  Demux1/2 -> Mux/2
  Demux1/1 -> Mux/1
  Fcn/1 -> Mux1/1
  Fcn1/1 -> Mux1/2
  Fcn2/1 -> Mux1/3

== system WF_onshore/VoltageSource/Subsystem1 ==
  v_abc : Inport
  Controlled Voltage Source : spsControlledVoltageSourceLib/Controlled Voltage Source  Initialize=on  Source_Type=AC  Amplitude=0  Phase=0  Frequency=0  Measurements=None
  Controlled Voltage Source1 : spsControlledVoltageSourceLib/Controlled Voltage Source  Initialize=on  Source_Type=AC  Amplitude=0  Phase=0  Frequency=0  Measurements=None
  Controlled Voltage Source2 : spsControlledVoltageSourceLib/Controlled Voltage Source  Initialize=on  Source_Type=AC  Amplitude=0  Phase=0  Frequency=0  Measurements=None
  Demux : Demux  Outputs=3
  Ground1 : spsGroundLib/Ground  LConnTagsString=a
  va : PMIOPort  Side=Right
  vb : PMIOPort  Port=2  Side=Right
  vc : PMIOPort  Port=3  Side=Right
  wires:
  Demux/1 -> Controlled Voltage Source/1
  Demux/2 -> Controlled Voltage Source1/1
  Demux/3 -> Controlled Voltage Source2/1
  v_abc/1 -> Demux/1
  connections:
  Controlled Voltage Source2/LConn1 -- Ground1/LConn1 -- Controlled Voltage Source1/LConn1 -- Controlled Voltage Source/LConn1
  va/RConn1 -- Controlled Voltage Source/RConn1
  vb/RConn1 -- Controlled Voltage Source1/RConn1
  vc/RConn1 -- Controlled Voltage Source2/RConn1

== system WF_onshore/VoltageSource/Subsystem2 ==
  x_d+ix_q : Inport
  Complex to Real-Imag2 : ComplexToRealImag
  Mux : Mux  Inputs=2
  x_dq : Outport
  wires:
  Complex to Real-Imag2/1 -> Mux/1
  Complex to Real-Imag2/2 -> Mux/2
  Mux/1 -> x_dq/1
  x_d+ix_q/1 -> Complex to Real-Imag2/1

== system WF_onshore/VoltageSource/grid inductance ==
  Series RLC Branch : spsSeriesRLCBranchLib/Series RLC Branch  LConnTagsString=__new0  RConnTagsString=__new0  BranchType=RL  Resistance=Rg+r_OH*Z_b_G  Inductance=(Lg+l_OH*(Z_b_G/(2*pi*f1)))  SetiL0=off  InitialCurrent=cvtr.ss.io0a  Capacitance=1e-6  Setx0=off  InitialVoltage=0  Measurements=None
  Series RLC Branch1 : spsSeriesRLCBranchLib/Series RLC Branch  LConnTagsString=__new0  RConnTagsString=__new0  BranchType=RL  Resistance=Rg+r_OH*Z_b_G  Inductance=(Lg+l_OH*(Z_b_G/(2*pi*f1)))  SetiL0=off  InitialCurrent=cvtr.ss.io0b  Capacitance=1e-6  Setx0=off  InitialVoltage=0  Measurements=None
  Series RLC Branch2 : spsSeriesRLCBranchLib/Series RLC Branch  LConnTagsString=__new0  RConnTagsString=__new0  BranchType=RL  Resistance=Rg+r_OH*Z_b_G  Inductance=(Lg+l_OH*(Z_b_G/(2*pi*f1)))  SetiL0=off  InitialCurrent=cvtr.ss.io0c  Capacitance=1e-6  Setx0=off  InitialVoltage=0  Measurements=None
  A : PMIOPort  Side=Left
  a : PMIOPort  Port=2  Side=Right
  B : PMIOPort  Port=3  Side=Left
  b : PMIOPort  Port=4  Side=Right
  C : PMIOPort  Port=5  Side=Left
  c : PMIOPort  Port=6  Side=Right
  connections:
  Series RLC Branch/RConn1 -- a/RConn1
  Series RLC Branch1/RConn1 -- b/RConn1
  Series RLC Branch2/RConn1 -- c/RConn1
  A/RConn1 -- Series RLC Branch/LConn1
  B/RConn1 -- Series RLC Branch1/LConn1
  C/RConn1 -- Series RLC Branch2/LConn1

== system WF_onshore/VoltageSource/grid inductance+line ==
  Constant : Constant  Value=Lg
  Series RLC Branch : spsSeriesRLCBranchLib/Series RLC Branch  LConnTagsString=__new0  RConnTagsString=__new0  BranchType=R  Resistance=Rg+r_OH*Z_b_G  Inductance=Lg  SetiL0=off  InitialCurrent=cvtr.ss.io0a  Capacitance=1e-6  Setx0=off  InitialVoltage=0  Measurements=None
  Series RLC Branch1 : spsSeriesRLCBranchLib/Series RLC Branch  LConnTagsString=__new0  RConnTagsString=__new0  BranchType=R  Resistance=Rg+r_OH*Z_b_G  Inductance=Lg  SetiL0=off  InitialCurrent=cvtr.ss.io0b  Capacitance=1e-6  Setx0=off  InitialVoltage=0  Measurements=None
  Series RLC Branch2 : spsSeriesRLCBranchLib/Series RLC Branch  LConnTagsString=__new0  RConnTagsString=__new0  BranchType=R  Resistance=Rg+r_OH*Z_b_G  Inductance=Lg  SetiL0=off  InitialCurrent=cvtr.ss.io0c  Capacitance=1e-6  Setx0=off  InitialVoltage=0  Measurements=None
  Step : Step  Time=0.2  Before=l_OH*(Z_b_G/(2*pi*f1))+Lg/10  After=l_OH*(Z_b_G/(2*pi*f1))+Lg  SampleTime=0
  Variable Inductor : spsVariableInductorLib/Variable Inductor  methode=Backward Euler  Labsmin=1e-6  Initialize=off  iL0=0  L0=1e-3  Vl0=0
      settings: LibrarySourceBlock=sps_lib/Passives/Variable Inductor
  Variable Inductor1 : spsVariableInductorLib/Variable Inductor  methode=Backward Euler  Labsmin=1e-6  Initialize=off  iL0=0  L0=1e-3  Vl0=0
      settings: LibrarySourceBlock=sps_lib/Passives/Variable Inductor
  Variable Inductor2 : spsVariableInductorLib/Variable Inductor  methode=Backward Euler  Labsmin=1e-6  Initialize=off  iL0=0  L0=1e-3  Vl0=0
      settings: LibrarySourceBlock=sps_lib/Passives/Variable Inductor
  A : PMIOPort  Side=Left
  a : PMIOPort  Port=2  Side=Right
  B : PMIOPort  Port=3  Side=Left
  b : PMIOPort  Port=4  Side=Right
  C : PMIOPort  Port=5  Side=Left
  c : PMIOPort  Port=6  Side=Right
  wires:
  Step/1 -> Variable Inductor/1, Variable Inductor2/1, Variable Inductor1/1
  connections:
  C/RConn1 -- Variable Inductor2/LConn1
  B/RConn1 -- Variable Inductor1/LConn1
  A/RConn1 -- Variable Inductor/LConn1
  Variable Inductor1/RConn1 -- Series RLC Branch1/LConn1
  Variable Inductor2/RConn1 -- Series RLC Branch2/LConn1
  Variable Inductor/RConn1 -- Series RLC Branch/LConn1
  Series RLC Branch/RConn1 -- a/RConn1
  Series RLC Branch1/RConn1 -- b/RConn1
  Series RLC Branch2/RConn1 -- c/RConn1
